simulink model "miniprojekt_state_space"  (R2020a)
settings: Solver=ode15s  StartTime=0.0  StopTime=10.0  RelTol=1e-3
values from neighbouring files (symbols this model uses):
  A = [(-c_p*ro_p*fp1-Kw)/Cvw, (c_p*ro_p*fp1)/Cvw; (c_p*ro_p*fp1)/Cvp, (-c_p*ro_p*fp1-Kp)/Cvp]    [statespace_transmitancja.m]    (also in statespace_transmitancja_leveled.m)
  B = [1/Cvw, Kw/Cvw; 0, Kp/Cvp]    [statespace_transmitancja.m]    (also in statespace_transmitancja_leveled.m)
  C = [1, 0; 0, 1]    [statespace_transmitancja.m]    (also in statespace_transmitancja_leveled.m)
  D = [0, 0; 0, 0]    [statespace_transmitancja.m]    (also in statespace_transmitancja_leveled.m)
  d_qg = 0    [nieliniowy.m]    (also in nieliniowy_leveled.m; statespace_transmitancja.m; statespace_transmitancja_leveled.m)
  d_Tzew = 2    [nieliniowy.m]    (also in nieliniowy_leveled.m; statespace_transmitancja.m; statespace_transmitancja_leveled.m)
  Init = [Twew0;Tp0]    [statespace_transmitancja.m]    (also in statespace_transmitancja_leveled.m)
  qg1 = 0.5*qgN    (= 750)    [nieliniowy.m]    (also in nieliniowy_leveled.m; statespace_transmitancja.m; statespace_transmitancja_leveled.m)
  Tzew1 = TzewN+5    (= 3)    [nieliniowy.m]    (also in nieliniowy_leveled.m; statespace_transmitancja.m; statespace_transmitancja_leveled.m)
settings Model: Creator=Jakub Szymkowiak  LastModifiedBy=Jakub Szymkowiak

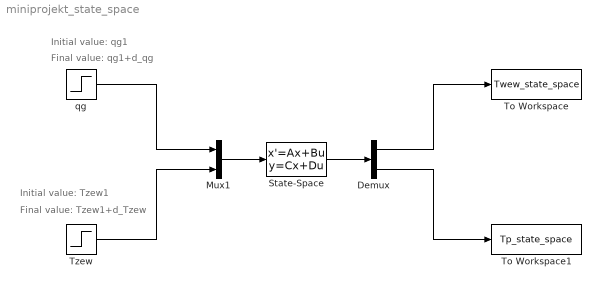
== system miniprojekt_state_space ==
  note: Final value: Tzew1+d_Tzew
  note: Initial value: Tzew1
  note: Final value: qg1+d_qg
  note: Initial value: qg1
  Demux : Demux  Outputs=2
  Mux1 : Mux  Inputs=2
  State-Space : StateSpace  A=A  B=B  C=C  D=D  InitialCondition=Init
  To Workspace : ToWorkspace  VariableName=Twew_state_space  SaveFormat=Timeseries  SampleTime=-1
  To Workspace1 : ToWorkspace  VariableName=Tp_state_space  SaveFormat=Timeseries  SampleTime=-1
  Tzew : Step  Before=Tzew1  After=Tzew1+d_Tzew  SampleTime=0
  qg : Step  Before=qg1  After=qg1+d_qg  SampleTime=0
  wires:
  qg/1 -> Mux1/1
  Tzew/1 -> Mux1/2
  Mux1/1 -> State-Space/1
  State-Space/1 -> Demux/1
  Demux/2 -> To Workspace1/1
  Demux/1 -> To Workspace/1
